simulink subsystem "ComputeErrors"  (R2023a)
settings: Solver=VariableStepAuto  StartTime=0.0  StopTime=10.0  RelTol=1e-3
settings Model: Creator=Andy  LastModifiedBy=Andy

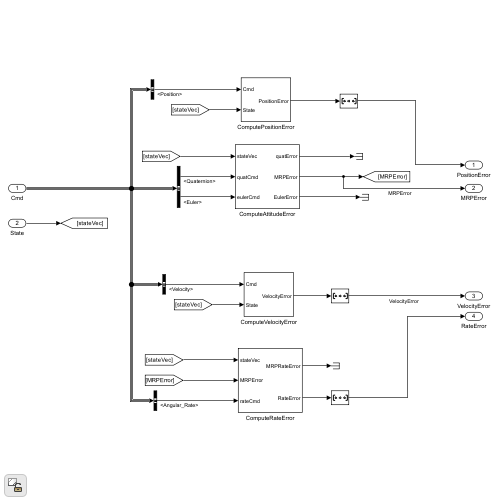
[thumbnail: Simulink's stored preview of the top-level diagram]
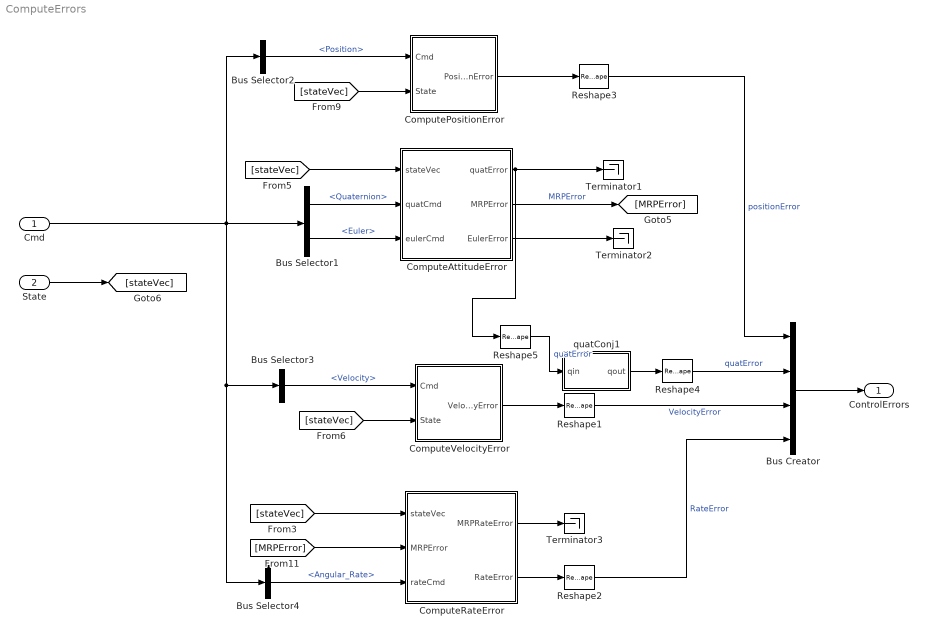
== system ComputeErrors ==
  Cmd : Inport
  State : Inport  Port=2
  Bus Creator : BusCreator  Inputs=4
  Bus Selector1 : BusSelector  OutputSignals=Quaternion,Euler
  Bus Selector2 : BusSelector  OutputSignals=Position
  Bus Selector3 : BusSelector  OutputSignals=Velocity
  Bus Selector4 : BusSelector  OutputSignals=Angular_Rate
  ComputeAttitudeError : Subsystem
  ComputePositionError : Subsystem
  ComputeRateError : Subsystem
  ComputeVelocityError : Subsystem
  Reshape{1..5} (5 alike) : Reshape  OutputDimensionality=Row vector (2-D)  OutputDimensions=[1,12]
  Terminator1 : Terminator
  Terminator2 : Terminator
  Terminator3 : Terminator
  quatConj1 : MATLAB Function  TreatAsAtomicUnit=on
  ControlErrors : Outport
  wires:
  Reshape5/1 -> quatConj1/1(qin)  "quatError"
  quatConj1/1(qout) -> Reshape4/1
  Reshape4/1 -> Bus Creator/2  "quatError"
  ComputeAttitudeError/1(quatError) -> Terminator1/1, Reshape5/1
  Bus Creator/1 -> ControlErrors/1
  State/1 -> [stateVec]
  Bus Selector4/1 -> ComputeRateError/3(rateCmd)  "<Angular_Rate>"
  Bus Selector3/1 -> ComputeVelocityError/1(Cmd)  "<Velocity>"
  Bus Selector2/1 -> ComputePositionError/1(Cmd)  "<Position>"
  Bus Selector1/1 -> ComputeAttitudeError/2(quatCmd)  "<Quaternion>"
  Reshape1/1 -> Bus Creator/3  "VelocityError"
  ComputeRateError/1(MRPRateError) -> Terminator3/1
  [MRPError] -> ComputeRateError/2(MRPError)
  ComputePositionError/1(PositionError) -> Reshape3/1
  ComputeRateError/2(RateError) -> Reshape2/1
  Bus Selector1/2 -> ComputeAttitudeError/3(eulerCmd)  "<Euler>"
  [stateVec] -> ComputeRateError/1(stateVec)
  Reshape2/1 -> Bus Creator/4  "RateError"
  [stateVec] -> ComputeAttitudeError/1(stateVec)
  [stateVec] -> ComputeVelocityError/2(State)
  ComputeVelocityError/1(VelocityError) -> Reshape1/1
  Cmd/1 -> Bus Selector2/1, Bus Selector1/1, Bus Selector3/1, Bus Selector4/1
  [stateVec] -> ComputePositionError/2(State)
  ComputeAttitudeError/3(EulerError) -> Terminator2/1
  Reshape3/1 -> Bus Creator/1  "positionError"
  ComputeAttitudeError/2(MRPError) -> [MRPError]  "MRPError"

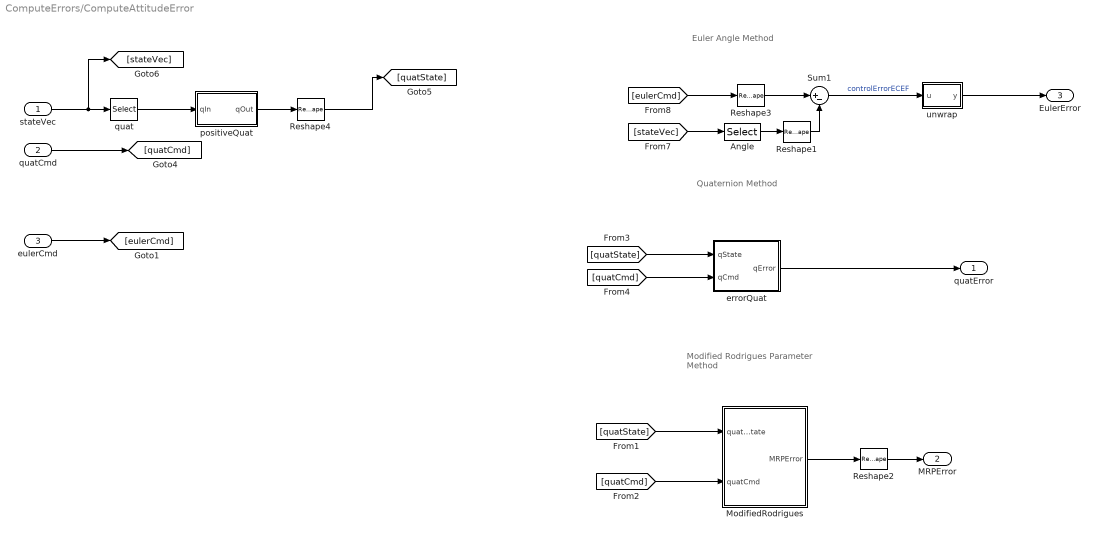
== system ComputeErrors/ComputeAttitudeError ==
  note: Quaternion Method
  note: Modified Rodrigues Parameter Method
  note: Euler Angle Method
  stateVec : Inport
  quatCmd : Inport  Port=2
  eulerCmd : Inport  Port=3
  Angle : Selector  IndexOptions=Index vector (dialog)  Indices=[4:6]  OutputSizes=1
  ModifiedRodrigues : Subsystem
  Reshape{1..4} (4 alike) : Reshape  OutputDimensionality=Row vector (2-D)  OutputDimensions=[1,12]
  Sum1 : Sum  Inputs=|+-
  errorQuat : MATLAB Function  TreatAsAtomicUnit=on
  positiveQuat : MATLAB Function  TreatAsAtomicUnit=on
  quat : Selector  IndexOptions=Index vector (dialog)  Indices=[13:16]  OutputSizes=1
  unwrap : MATLAB Function  TreatAsAtomicUnit=on
  quatError : Outport
  MRPError : Outport  Port=2
  EulerError : Outport  Port=3
  wires:
  positiveQuat/1(qOut) -> Reshape4/1
  [quatState] -> errorQuat/1(qState)
  stateVec/1 -> [stateVec], quat/1
  errorQuat/1(qError) -> quatError/1
  [quatCmd] -> errorQuat/2(qCmd)
  quat/1 -> positiveQuat/1(qIn)
  quatCmd/1 -> [quatCmd]
  [quatState] -> ModifiedRodrigues/1(quatState)
  [quatCmd] -> ModifiedRodrigues/2(quatCmd)
  eulerCmd/1 -> [eulerCmd]
  ModifiedRodrigues/1(MRPError) -> Reshape2/1
  [stateVec] -> Angle/1
  [eulerCmd] -> Reshape3/1
  Angle/1 -> Reshape1/1
  Sum1/1 -> unwrap/1(u)  "controlErrorECEF"
  unwrap/1(y) -> EulerError/1
  Reshape4/1 -> [quatState]
  Reshape1/1 -> Sum1/2
  Reshape2/1 -> MRPError/1
  Reshape3/1 -> Sum1/1

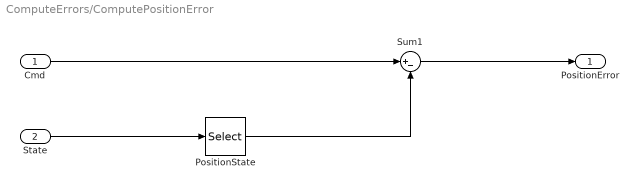
== system ComputeErrors/ComputePositionError ==
  Cmd : Inport
  State : Inport  Port=2
  PositionState : Selector  IndexOptions=Index vector (dialog)  Indices=[1:3]  OutputSizes=1
  Sum1 : Sum  Inputs=|+-
  PositionError : Outport
  wires:
  State/1 -> PositionState/1
  Sum1/1 -> PositionError/1
  PositionState/1 -> Sum1/2
  Cmd/1 -> Sum1/1

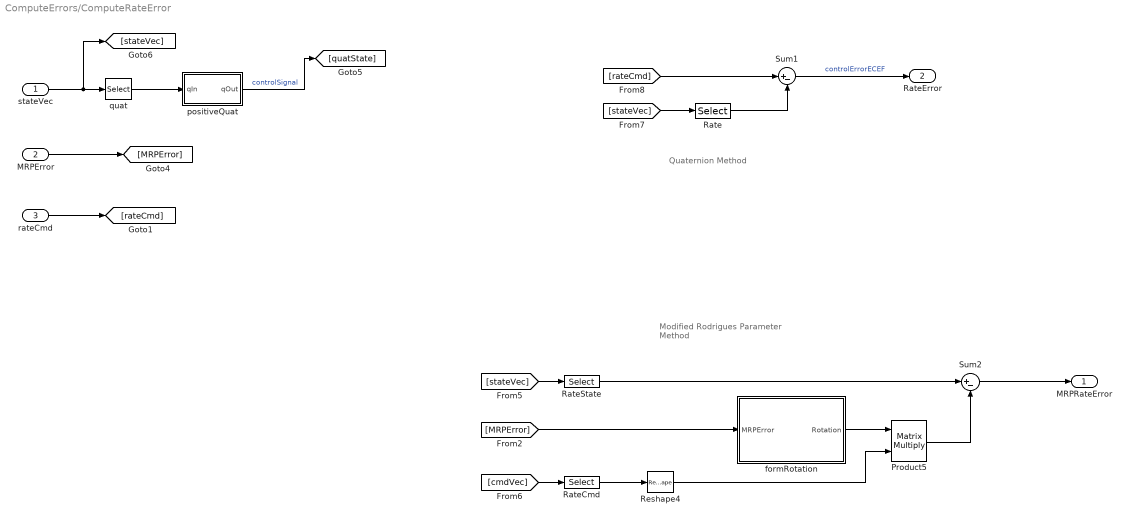
== system ComputeErrors/ComputeRateError ==
  note: Modified Rodrigues Parameter Method
  note: Quaternion Method
  stateVec : Inport
  MRPError : Inport  Port=2
  rateCmd : Inport  Port=3
  Product5 : Product  Multiplication=Matrix(*)
  Rate : Selector  IndexOptions=Index vector (dialog)  Indices=[10:12]  OutputSizes=1
  RateCmd : Selector  IndexOptions=Index vector (dialog)  Indices=[10:12]  OutputSizes=1
  RateState : Selector  IndexOptions=Index vector (dialog)  Indices=[10:12]  OutputSizes=1
  Reshape4 : Reshape  OutputDimensionality=Column vector (2-D)  OutputDimensions=[1,12]
  Sum1 : Sum  Inputs=|+-
  Sum2 : Sum  Inputs=|+-
  formRotation : MATLAB Function  TreatAsAtomicUnit=on
  positiveQuat : MATLAB Function  TreatAsAtomicUnit=on
  quat : Selector  IndexOptions=Index vector (dialog)  Indices=[13:16]  OutputSizes=1
  MRPRateError : Outport
  RateError : Outport  Port=2
  wires:
  Sum1/1 -> RateError/1  "controlErrorECEF"
  Rate/1 -> Sum1/2
  [rateCmd] -> Sum1/1
  [stateVec] -> Rate/1
  Sum2/1 -> MRPRateError/1
  rateCmd/1 -> [rateCmd]
  [cmdVec] -> RateCmd/1
  RateCmd/1 -> Reshape4/1
  [stateVec] -> RateState/1
  MRPError/1 -> [MRPError]
  quat/1 -> positiveQuat/1(qIn)
  stateVec/1 -> quat/1, [stateVec]
  positiveQuat/1(qOut) -> [quatState]  "controlSignal"
  RateState/1 -> Sum2/1
  formRotation/1(Rotation) -> Product5/1
  Product5/1 -> Sum2/2
  Reshape4/1 -> Product5/2
  [MRPError] -> formRotation/1(MRPError)

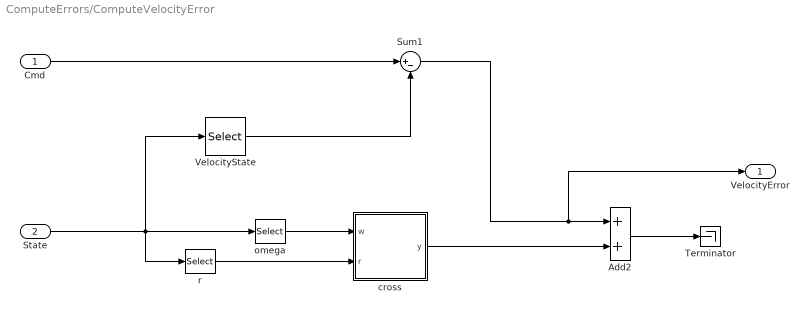
== system ComputeErrors/ComputeVelocityError ==
  Cmd : Inport
  State : Inport  Port=2
  Add2 : Sum
  Sum1 : Sum  Inputs=|+-
  Terminator : Terminator
  VelocityState : Selector  IndexOptions=Index vector (dialog)  Indices=[7:9]  OutputSizes=1
  cross : MATLAB Function  TreatAsAtomicUnit=on
  omega : Selector  IndexOptions=Index vector (dialog)  Indices=[10:12]  OutputSizes=1
  r : Selector  IndexOptions=Index vector (dialog)  Indices=[1:3]  OutputSizes=1
  VelocityError : Outport
  wires:
  Add2/1 -> Terminator/1
  State/1 -> VelocityState/1, r/1, omega/1
  cross/1(y) -> Add2/2
  omega/1 -> cross/1(w)
  Sum1/1 -> Add2/1, VelocityError/1
  r/1 -> cross/2(r)
  VelocityState/1 -> Sum1/2
  Cmd/1 -> Sum1/1

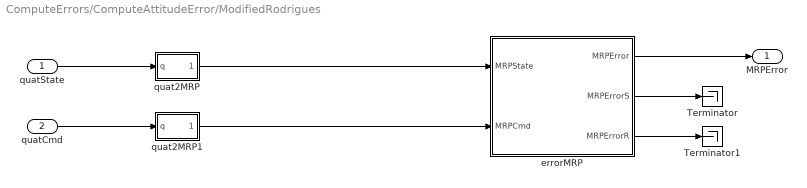
== system ComputeErrors/ComputeAttitudeError/ModifiedRodrigues ==
  quatState : Inport
  quatCmd : Inport  Port=2
  Terminator : Terminator
  Terminator1 : Terminator
  errorMRP : MATLAB Function  TreatAsAtomicUnit=on
  quat2MRP : MATLAB Function  TreatAsAtomicUnit=on
  quat2MRP1 : MATLAB Function  TreatAsAtomicUnit=on
  MRPError : Outport
  wires:
  errorMRP/3(MRPErrorR) -> Terminator1/1
  errorMRP/2(MRPErrorS) -> Terminator/1
  quatState/1 -> quat2MRP/1(q)
  errorMRP/1(MRPError) -> MRPError/1
  quat2MRP/1(mrp) -> errorMRP/1(MRPState)
  quat2MRP1/1(mrp) -> errorMRP/2(MRPCmd)
  quatCmd/1 -> quat2MRP1/1(q)

== matlab function ComputeErrors/ComputeAttitudeError/ModifiedRodrigues/errorMRP ==
  data: MRPError output; MRPState input; MRPCmd input; MRPErrorS output; MRPErrorR output
function [MRPError, MRPErrorS, MRPErrorR]   = callcomputeErrorMRP(MRPState,MRPCmd)

% Reference:  Shuster, Malcolm D. "A survey of attitude representations." Navigation 8, no. 9 (1993): 439-517.

% Error formed by MRP composition operator Ref. 1, Eq. 257 
% Cmd comp State

% Compute the square of the norm for each MRP
normSqrdState = norm(MRPState)^2;
normSqrdCmd = norm(MRPCmd)^2;

% Compute MRP error
num = (1 - normSqrdState)*MRPCmd - (1 - normSqrdCmd)*MRPState - 2*skewMat(MRPCmd)*MRPState;
den = 1 + normSqrdCmd*normSqrdState - 2*MRPCmd'*MRPState;

MRPError = num/den;
% MRPError(3) = -1*MRPError(3);

MRPErrorR = MRPError;
% Compute error using shadow set of MRP
MRPStateS = -MRPState / (dot(MRPState',MRPState));
normSqrdStateS = norm(MRPStateS)^2;
numS = (1 - normSqrdStateS)*MRPCmd - (1 - normSqrdCmd)*MRPStateS - 2*skewMat(MRPCmd)*MRPStateS;
denS = 1 + normSqrdCmd*normSqrdStateS - 2*MRPCmd'*MRPStateS;
MRPErrorS = numS/denS;


if norm(MRPState) > 1e-3
    % Compute error using shadow set of MRP
    MRPStateS = -MRPState / (dot(MRPState',MRPState));
    normSqrdStateS = norm(MRPStateS)^2;
    numS = (1 - normSqrdStateS)*MRPCmd - (1 - normSqrdCmd)*MRPStateS - 2*skewMat(MRPCmd)*MRPStateS;
    denS = 1 + normSqrdCmd*normSqrdStateS - 2*MRPCmd'*MRPStateS;
    MRPErrorS = numS/denS;

    % Use the smallest error value between the originial MPR and shadow set
    if norm(MRPErrorS) < norm(MRPError)
        MRPError = MRPErrorS;
    end
end

% s = dot(MRPError',MRPError);
% if s > 0.98 && s < 1.02
%     MRPError = -MRPError/s;
% end
MRPError = MRPCmd - MRPState;
MRPErrorR = MRPError;

if norm(MRPCmd) > 1/3
    % Compute error using shadow set of MRP
    MRPCmdS = -MRPCmd / (dot(MRPCmd',MRPCmd));
    MRPErrorS = MRPCmdS - MRPState;

    % Use the smallest error value between the originial MPR and shadow set
    if norm(MRPErrorS) < norm(MRPError)
        MRPError = MRPErrorS;
    end
end

== matlab function ComputeErrors/ComputeAttitudeError/ModifiedRodrigues/quat2MRP ==
  data: mrp output; q input
function mrp   = callquatToMRP(q)

[mrp] = quatToMRP(q);

== matlab function ComputeErrors/ComputeAttitudeError/ModifiedRodrigues/quat2MRP1 ==
  data: mrp output; q input
function mrp  = callquatToMRP(q)

[mrp] = quatToMRP(q);

== matlab function ComputeErrors/ComputeAttitudeError/errorQuat ==
  data: qError output; qState input; qCmd input
function qError   = callcomputeErrorQuaternion(qState,qCmd)

%qError = qState;
if qState(1) < 0
    qState = -1.*qState;
end
if qCmd(1) < 0
    qCmd = -1.*qCmd;
end

[qError] = computeErrorQuaternion(qState,quatconj(qCmd))';

== matlab function ComputeErrors/ComputeAttitudeError/positiveQuat ==
  data: qOut output; qIn input
function qOut  = positiveQat(qIn)


if qIn(1) < 0
    qOut = -1.*qIn;
else
    qOut = qIn;
end

== matlab function ComputeErrors/ComputeAttitudeError/unwrap ==
  data: y output; u input
function y  = fcn(u)


y = unwrap(u);

== matlab function ComputeErrors/ComputeRateError/formRotation ==
  data: Rotation output; MRPError input
function Rotation  = callcomputeBodyRotation(MRPError)

skewError = skewMat(MRPError);
nsqError = norm(MRPError)^2;
Rotation = eye(3,3) + (8*skewError*skewError - 4*(1 - nsqError)*skewError)*(1+nsqError)^(-2);

== matlab function ComputeErrors/ComputeRateError/positiveQuat ==
  data: qOut output; qIn input
function qOut  = positiveQat(qIn)


if qIn(1) < 0
    qOut = -1.*qIn;
else
    qOut = qIn;
end

== matlab function ComputeErrors/ComputeVelocityError/cross ==
  data: y output; w input; r input
function y  = fcn(w,r)


y = cross(w,r);

== matlab function ComputeErrors/quatConj1 ==
  data: qin input; qout output
function qout  = callquatconj(qin)

[qout] = quatconj(qin);
